simulink model "robot"  (R2022b)
settings: Solver=VariableStepAuto  StartTime=0.0  StopTime=20  MaxStep=0.01  RelTol=1e-3
settings Model: Creator=mathe  LastModifiedBy=mathe

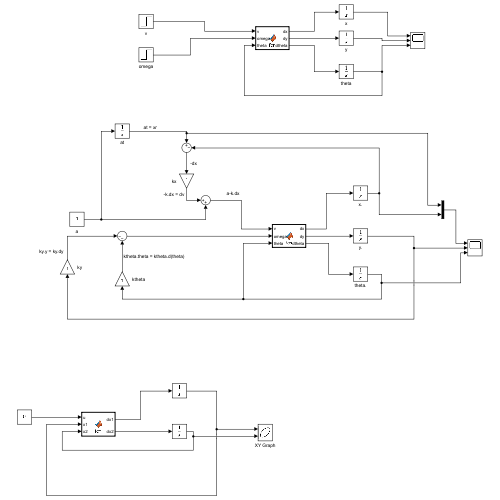
[thumbnail: Simulink's stored preview of the top-level diagram]
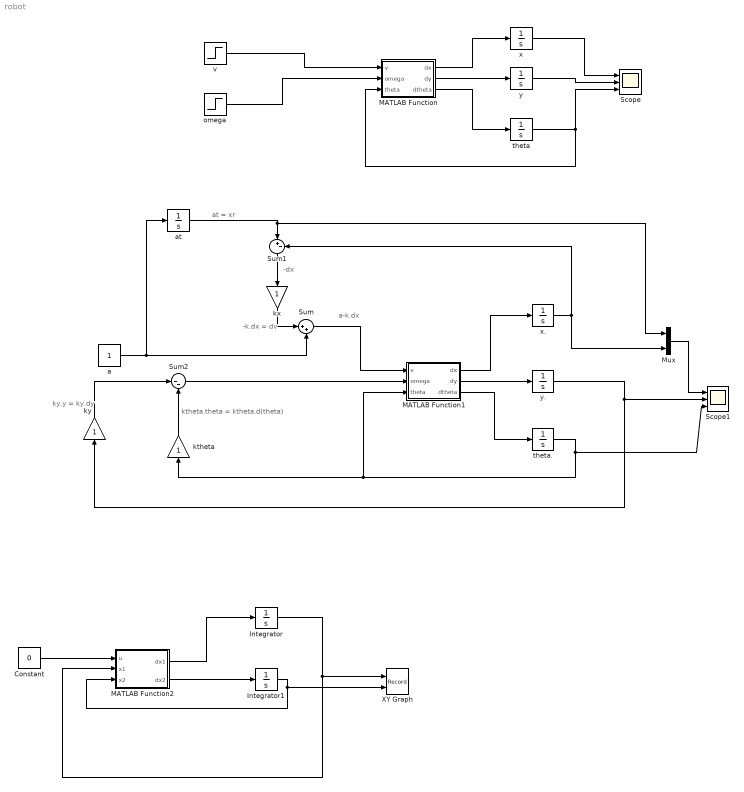
== system robot ==
  note: ky.y = ky.dy
  note: ktheta.theta = ktheta.d(theta)
  note: a-k.dx
  note: -k.dx = dv
  note: -dx
  note: at = xr
  Constant : Constant  Value=0
  Integrator : Integrator  InitialCondition=1
  Integrator1 : Integrator  InitialCondition=0.4
  MATLAB Function : MATLAB Function  TreatAsAtomicUnit=on
  MATLAB Function1 : MATLAB Function  TreatAsAtomicUnit=on
  MATLAB Function2 : MATLAB Function  TreatAsAtomicUnit=on
  Mux : Mux  Inputs=2
  Scope : Scope  NumInputPorts=3
  Scope1 : Scope  NumInputPorts=3
  Sum : Sum  Inputs=|++
  Sum1 : Sum  Inputs=|+-
  Sum2 : Sum  Inputs=|--
  XY Graph : Record  FileSettingsInternal="{\"entries\":[{\"content\":{\"excelSettings\":{\"content\":{},\"type\":\"Streamout.ExcelSettings\"}},\"type\":\"Streamout.FileSettingStorage\",\"uuid\":\"fc4d958a-e6ba-42b8-865c-33b7ea9480a9\"}],\"packageUris\":[\"http://schema.mathworks.com/mf0/streamout_blocks/R2020a\"],\"version\":\"1.0\"}"  Layout=[1 1]  SignalsInternal="{\"entries\":[{\"content\":{\"signals\":[{\"content\":{\"blockPath\":[\"robot/XY Graph\"],\"channel\":[],\"dimensions\":[1],\"domain\":\"robot/XY Graph\",\"lineColor\":\"#a2142f\",\"plots\":[1],\"port\":1,\"sid\":[\"\"],\"signalID\":35,\"signalName\":\"Integrator\"},\"type\":\"RecordBlkView.Signal\",\"uuid\":\"0225e2f5-7c19-43f5-a54d-7a91d70c9435\"},{\"content\":{\"blockPath\":[\"robot/XY Graph\"],\"channel\":[],\"dimensions\":[1],\"domain\":\"robot/XY Graph\",\"lineColor\":\"#139fff\",\"plots\":[1],\"port\":2,\"sid\":[\"\"],\"signalID\":39,\"signalName\":\"Integrator1\"},\"type\":\"RecordBlkView.Signal\",\"uuid\":\"c80e7c24-8514-49b2-8fc5-971aafed3c48\"}]},\"type\":\"RecordBlkView.InputSignals\",\"uuid\":\"eb2e0804-cebb-4b0e-b699-18a626d001db\"}],\"packageUris\":[\"http://schema.mathworks.com/mf0/streamout_blocks/R2020a\"],\"version\":\"1.0\"}"  VisualizationBindings="{\"xyplotplugin\":{\"info\":[{\"series\":[{\"bindingParametersList\":[{\"parameter\":\"X-Axis\",\"signalID\":35,\"signalName\":\"Integrator\"},{\"parameter\":\"Y-Axis\",\"signalID\":39,\"signalName\":\"Integrator1\"}],\"seriesID\":26402}],\"subplotID\":1}]}}"  CompatibilityTag=XY  st=-1
  a : Constant
  at : Integrator
  ktheta : Gain
  kx : Gain
  ky : Gain
  omega : Step  SampleTime=3
  theta : Integrator
  theta. : Integrator  InitialCondition=0.1
  v : Step  SampleTime=3
  x : Integrator
  x. : Integrator  InitialCondition=1
  y : Integrator
  y. : Integrator  InitialCondition=0.1
  wires:
  MATLAB Function/1(dx) -> x/1
  MATLAB Function/2(dy) -> y/1
  MATLAB Function/3(dtheta) -> theta/1
  x/1 -> Scope/1
  y/1 -> Scope/2
  theta/1 -> Scope/3, MATLAB Function/3(theta)
  v/1 -> MATLAB Function/1(v)
  omega/1 -> MATLAB Function/2(omega)
  MATLAB Function1/1(dx) -> x./1
  MATLAB Function1/2(dy) -> y./1
  MATLAB Function1/3(dtheta) -> theta./1
  x./1 -> Mux/2, Sum1/2
  Sum1/1 -> kx/1
  Sum/1 -> MATLAB Function1/1(v)
  kx/1 -> Sum/1
  a/1 -> Sum/2, at/1
  at/1 -> Mux/1, Sum1/1
  Sum2/1 -> MATLAB Function1/2(omega)
  ktheta/1 -> Sum2/2
  ky/1 -> Sum2/1
  theta./1 -> MATLAB Function1/3(theta), ktheta/1, Scope1/3
  y./1 -> Scope1/2, ky/1
  Mux/1 -> Scope1/1
  Constant/1 -> MATLAB Function2/1(u)
  MATLAB Function2/1(dx1) -> Integrator/1
  Integrator/1 -> XY Graph/1, MATLAB Function2/2(x1)
  MATLAB Function2/2(dx2) -> Integrator1/1
  Integrator1/1 -> XY Graph/2, MATLAB Function2/3(x2)

== matlab function robot/MATLAB Function1 ==
  data: v input; dx output; omega input; theta input; dy output; dtheta output
function [dx, dy, dtheta] = fcn(v, omega, theta)

dx = v*cos(theta);
dy = v*sin(theta);
dtheta = omega;

== matlab function robot/MATLAB Function ==
  data: v input; dx output; omega input; theta input; dy output; dtheta output
function [dx, dy, dtheta] = fcn(v, omega, theta)

dx = v*cos(theta);
dy = v*sin(theta);
dtheta = omega;

== matlab function robot/MATLAB Function2 ==
  data: u input; x1 input; dx1 output; x2 input; dx2 output
function [dx1, dx2] = fcn(u, x1, x2)

rho = 1;
dx1 = x2;
dx2 = -rho*(x1^2-1)*x2 - x1 + u;
